simulink model "problem4"  (R2024b)
settings: Solver=VariableStepAuto  StartTime=0.0  StopTime=1000  RelTol=1e-3
values from neighbouring files (symbols this model uses):
  alpha = [1.922E-4, 1.847E-4]    [problem4_constants.m]    (also in problem4_setup.m = [1.847E-4; 1.922E-4])
  beta = [1, -1.8850, 0.8869]    [problem4_constants.m]    (also in problem4_setup.m = [0.8869; -1.8850])
  lambda = 1    [problem3.m]    (also in problem3_constants.m; problem3_setup.m; problem4_constants.m)
  P0 = 1 * eye(2)    [problem3.m]    (also in problem3_constants.m = 100 * eye(2); problem3_setup.m = 1000 * eye(2); problem4_setup.m = 100 * eye(4))
settings Model: Creator=djd14  LastModifiedBy=djd14

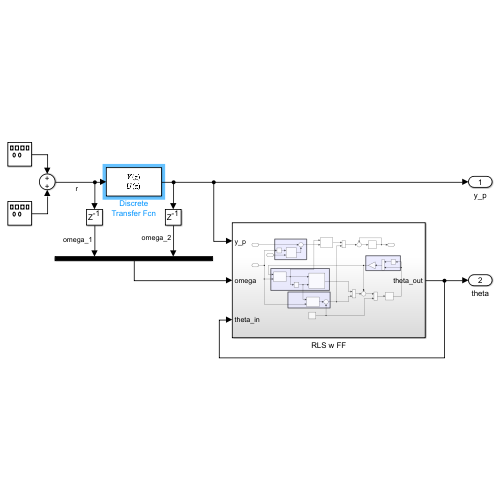
[thumbnail: Simulink's stored preview of the top-level diagram]
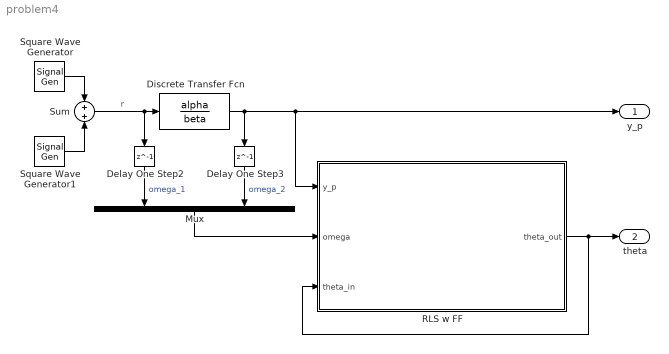
== system problem4 ==
  Delay One Step2 : Delay  DelayLength=1
  Delay One Step3 : Delay  DelayLength=1
  Discrete Transfer Fcn : DiscreteTransferFcn  Numerator=alpha  Denominator=beta
  Mux : Mux  Inputs=2
  RLS w FF : Subsystem
  Square Wave Generator : SignalGenerator  WaveForm=square  Frequency=0.02  Units=rad/sec
  Square Wave Generator1 : SignalGenerator  WaveForm=square  Frequency=0.1  Units=rad/sec
  Sum : Sum  Inputs=+|+
  y_p : Outport
  theta : Outport  Port=2
  wires:
  Delay One Step2/1 -> Mux/1  "omega_1"
  RLS w FF/1(theta_out) -> theta/1, RLS w FF/3(theta_in)
  Sum/1 -> Discrete Transfer Fcn/1, Delay One Step2/1  "r"
  Delay One Step3/1 -> Mux/2  "omega_2"
  Mux/1 -> RLS w FF/2(omega)
  Discrete Transfer Fcn/1 -> y_p/1, RLS w FF/1(y_p), Delay One Step3/1
  Square Wave Generator1/1 -> Sum/2
  Square Wave Generator/1 -> Sum/1

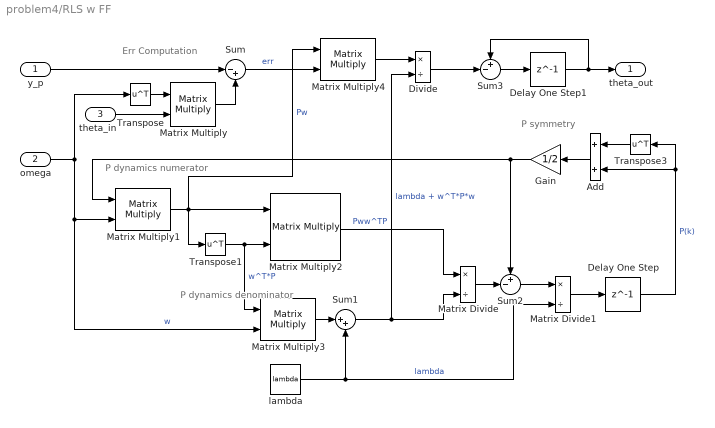
== system problem4/RLS w FF ==
  note: P symmetry
  note: P dynamics denominator
  note: P dynamics numerator
  note: Err Computation
  y_p : Inport
  omega : Inport  Port=2
  theta_in : Inport  Port=3
  Add : Sum
  Delay One Step : Delay  DelayLength=1  InitialCondition=P0
  Delay One Step1 : Delay  DelayLength=1
  Divide : Product  Inputs=*/
  Gain : Gain  Gain=1/2
  Matrix Divide : Product  Inputs=*/
  Matrix Divide1 : Product  Inputs=*/
  Matrix Multiply{,1..4} (5 alike) : Product  Multiplication=Matrix(*)
  Sum : Sum  Inputs=|-+
  Sum1 : Sum  Inputs=|++
  Sum2 : Sum  Inputs=+-|
  Sum3 : Sum  Inputs=+-|
  Transpose : Math  Operator=transpose
  Transpose1 : Math  Operator=transpose
  Transpose3 : Math  Operator=transpose
  lambda : Constant  Value=lambda
  theta_out : Outport
  wires:
  omega/1 -> Transpose/1, Matrix Multiply3/2, Matrix Multiply1/2  "w"
  theta_in/1 -> Matrix Multiply/2
  Transpose/1 -> Matrix Multiply/1
  y_p/1 -> Sum/1
  Matrix Multiply/1 -> Sum/2
  Sum/1 -> Matrix Multiply4/2  "err"
  Matrix Multiply1/1 -> Matrix Multiply4/1, Matrix Multiply2/1, Transpose1/1  "Pw"
  Delay One Step/1 -> Transpose3/1, Add/2  "P(k)"
  Matrix Multiply2/1 -> Matrix Divide/1  "Pww^TP"
  Transpose1/1 -> Matrix Multiply3/1, Matrix Multiply2/2  "w^T*P"
  Matrix Multiply3/1 -> Sum1/1
  Sum1/1 -> Divide/2, Matrix Divide/2  "lambda + w^T*P*w"
  Matrix Divide/1 -> Sum2/2
  Sum2/1 -> Matrix Divide1/1
  Matrix Divide1/1 -> Delay One Step/1
  Transpose3/1 -> Add/1
  Add/1 -> Gain/1
  Gain/1 -> Matrix Multiply1/1, Sum2/1
  lambda/1 -> Matrix Divide1/2, Sum1/2  "lambda"
  Sum3/1 -> Delay One Step1/1
  Delay One Step1/1 -> theta_out/1, Sum3/1
  Matrix Multiply4/1 -> Divide/1
  Divide/1 -> Sum3/2
